simulink model "model2v7"  (R2020b)
settings: Solver=VariableStepAuto  StartTime=0.0  StopTime=10.0  RelTol=1e-3
settings Model: Creator=dkravchenko  LastModifiedBy=dkravchenko

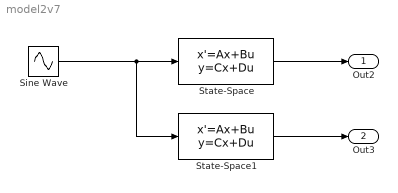
== system model2v7 ==
  Sine Wave : Sin  Amplitude=0  Bias=1  Frequency=0  SampleTime=0
  State-Space : StateSpace  A=[1 2; -10 -3]  B=[0; 1]  C=[8 2]  D=0  InitialCondition=0
  State-Space1 : StateSpace  A=[1 2; -10 -3]  B=[0; -1]  C=[-8 -2]  D=0  InitialCondition=0
  Out2 : Outport
  Out3 : Outport  Port=2
  wires:
  State-Space1/1 -> Out3/1
  Sine Wave/1 -> State-Space1/1, State-Space/1
  State-Space/1 -> Out2/1
